simulink model "PWM_3_Phase_Inverter"  (R2024b)
settings: Solver=ode3  StartTime=0.0  StopTime=0.01  FixedStep=10e-6  RelTol=1e-3
libraries: spsIGBTLib x6, simulink x3, spsDCVoltageSourceLib x1, spsGroundLib x1, spsSawtoothGeneratorLib x1, spsThreePhaseParallelRLCBranchLib x1, spsThreePhaseVIMeasurementLib x1, sps_lib x1
settings Model: Creator=PRASHANTH  LastModifiedBy=PRASHANTH

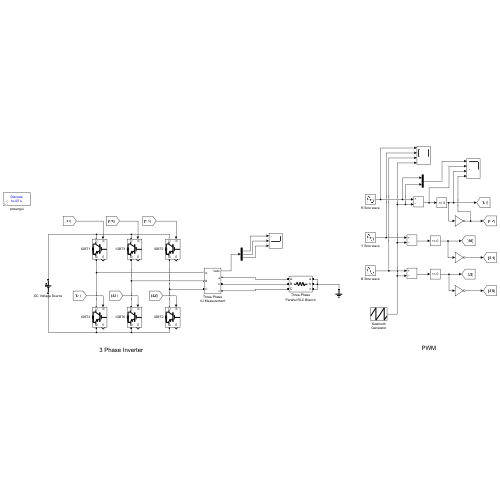
[thumbnail: Simulink's stored preview of the top-level diagram]
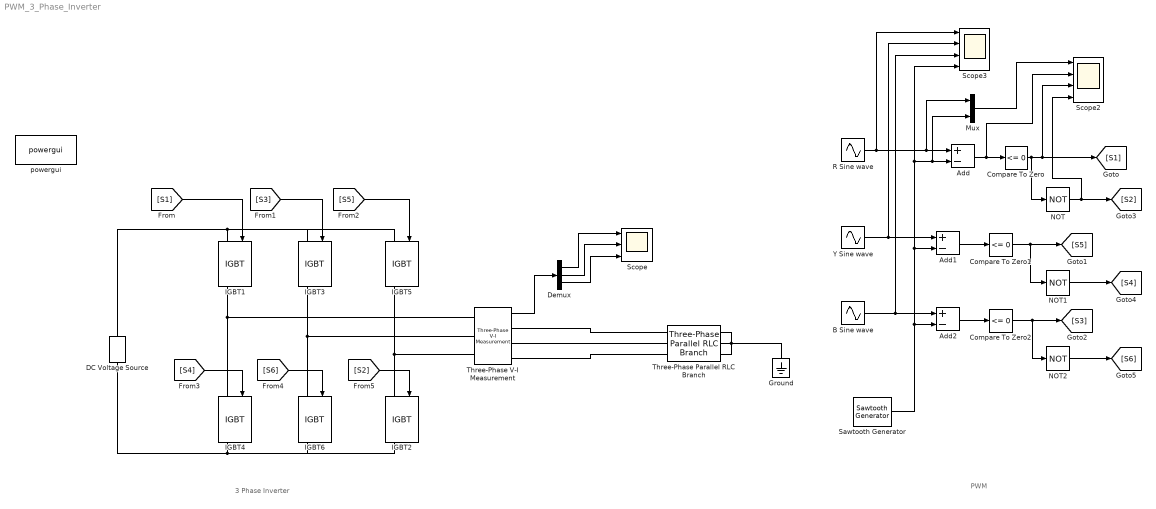
== system PWM_3_Phase_Inverter ==
  note: PWM
  note: 3 Phase Inverter
  Add : Sum  Inputs=+-
  Add1 : Sum  Inputs=+-
  Add2 : Sum  Inputs=+-
  B Sine wave : Sin  Frequency=round(2*pi*50,5)  Phase=round(-2*pi/3,5)  SampleTime=0
  Compare To Zero : simulink/Logic and Bit Operations/Compare To Zero  relop=<=  OutDataTypeStr=boolean
  Compare To Zero1 : simulink/Logic and Bit Operations/Compare To Zero  relop=<=  OutDataTypeStr=boolean
  Compare To Zero2 : simulink/Logic and Bit Operations/Compare To Zero  relop=<=  OutDataTypeStr=boolean
  DC Voltage Source : spsDCVoltageSourceLib/DC Voltage Source  Amplitude=460/sqrt(3)  Measurements=None
  Demux : Demux  Outputs=3
  Ground : spsGroundLib/Ground  LConnTagsString=a
  IGBT{1..6} (6 alike) : spsIGBTLib/IGBT  Ron=0.001  Lon=0  Vf=1  Tf=1e-6  Tt=2e-6  IC=0  Rs=1e5  Cs=inf  Measurements=on
  Mux : Mux  Inputs=2
  NOT : Logic  Operator=NOT  IconShape=distinctive  AllPortsSameDT=off  OutDataTypeStr=boolean
  NOT1 : Logic  Operator=NOT  IconShape=distinctive  AllPortsSameDT=off  OutDataTypeStr=boolean
  NOT2 : Logic  Operator=NOT  IconShape=distinctive  AllPortsSameDT=off  OutDataTypeStr=boolean
  R Sine wave : Sin  Frequency=round(2*pi*50,5)  SampleTime=0
  Sawtooth Generator : spsSawtoothGeneratorLib/Sawtooth Generator  Freq=10e3  Phase=120  Ts=0
  Scope : Scope  NumInputPorts=3
  Scope2 : Scope  NumInputPorts=4
  Scope3 : Scope  NumInputPorts=4
  Three-Phase Parallel RLC Branch : spsThreePhaseParallelRLCBranchLib/Three-Phase Parallel RLC Branch  LConnTagsString=A|B|C  RConnTagsString=A|B|C  BranchType=R  Resistance=1  Inductance=1e-3  Capacitance=1e-6  Measurements=None
  Three-Phase V-I Measurement : spsThreePhaseVIMeasurementLib/Three-Phase V-I Measurement  VoltageMeasurement=phase-to-ground  SetLabelV=off  LabelV=Vabc  Vpu=off  VpuLL=off  CurrentMeasurement=no  SetLabelI=off  LabelI=Iabc  Ipu=off  Pbase=100e6  Vbase=500e3  OutputType=Complex  PhasorSimulation=off  PSBequivalent=0
  Y Sine wave : Sin  Frequency=round(2*pi*50,5)  Phase=round(2*pi/3,5)  SampleTime=0
  powergui : sps_lib/powergui  Priority=1  SimulationMode=Discrete  SampleTime=10e-6  frequency=60  Iterations=50  frequencyindice=0  Pbase=100e6  ErrMax=1e-4  UnitsV=kV  UnitsW=MW  buscounter=0  FunctionMessages=off  echomessages=off  EnableUseOfTLC=off  CurrentSourceSwitches=off  DisableSnubberDevices=off  DisableRonSwitches=off  DisableVfSwitches=off  DisplayEquations=off  AutomaticDiscreteSolvers=off  SolverType=Tustin/Backward Euler (TBE)  Interpol=off  ExternalGateDelay=off  methode=off  Ts=100  x0status=blocks  SPID=on  SwTol=0  HookPort=off  NonlinearTolerance=1e-4  nMaxIteration=100  ContinueOnMaxIteration=off  RestoreLinks=warning  ResistiveCurrentMeasurement=off  Frange=[0:2:500]  Ylog=off  Xlog=on  ShowGrid=off  save=off  variable=ZData  structure=0  ZoomFFT=off  StartTime=0.0  cycles=1  DisplayStyle=1  fundamental=60  FreqAxis=off  MaxFrequency=1000  frequencyindicesteady=1  RmsSteady=1  display=off
  wires:
  Y Sine wave/1 -> Scope3/2, Add1/1
  R Sine wave/1 -> Scope3/1, Add/1, Mux/1
  Add2/1 -> Compare To Zero2/1
  Add1/1 -> Compare To Zero1/1
  Add/1 -> Scope2/2, Compare To Zero/1
  Compare To Zero2/1 -> NOT2/1, [S3]
  Compare To Zero1/1 -> NOT1/1, [S5]
  Compare To Zero/1 -> NOT/1, Scope2/3, [S1]
  NOT/1 -> Scope2/4, [S2]
  NOT1/1 -> [S4]
  NOT2/1 -> [S6]
  [S1] -> IGBT1/1
  [S3] -> IGBT3/1
  [S5] -> IGBT5/1
  [S4] -> IGBT4/1
  [S6] -> IGBT6/1
  [S2] -> IGBT2/1
  Three-Phase V-I Measurement/1 -> Demux/1
  Demux/1 -> Scope/1
  Demux/2 -> Scope/2
  Demux/3 -> Scope/3
  Sawtooth Generator/1 -> Scope3/4, Mux/2, Add/2, Add1/2, Add2/2
  Mux/1 -> Scope2/1
  B Sine wave/1 -> Scope3/3, Add2/1
  connections:
  DC Voltage Source/RConn1 -- IGBT5/LConn1 -- IGBT3/LConn1 -- IGBT1/LConn1
  DC Voltage Source/LConn1 -- IGBT2/RConn1 -- IGBT6/RConn1 -- IGBT4/RConn1
  IGBT1/RConn1 -- Three-Phase V-I Measurement/LConn1 -- IGBT4/LConn1
  IGBT3/RConn1 -- Three-Phase V-I Measurement/LConn2 -- IGBT6/LConn1
  IGBT5/RConn1 -- IGBT2/LConn1 -- Three-Phase V-I Measurement/LConn3
  Three-Phase V-I Measurement/RConn1 -- Three-Phase Parallel RLC Branch/LConn1
  Three-Phase Parallel RLC Branch/LConn2 -- Three-Phase V-I Measurement/RConn2
  Three-Phase Parallel RLC Branch/LConn3 -- Three-Phase V-I Measurement/RConn3
  Three-Phase Parallel RLC Branch/RConn1 -- Ground/LConn1 -- Three-Phase Parallel RLC Branch/RConn2 -- Three-Phase Parallel RLC Branch/RConn3
